simulink model "rate_feedforward_test"  (R2018b)
settings: Solver=FixedStepAuto  StartTime=0.0  StopTime=600  FixedStep=simParams.sample_time_s  RelTol=1e-3
undefined symbols (not defined in the file): simParams
libraries: aerolibutil x2, simulink x1, vrlib x1, clock_lib x1, groundpass_predict_lib x1, sgp4_lib_fsw x1, sunVectorEclipse_lib x1, time_coord_rotations_lib x1, target_gen_lib x1
settings Model: Creator=Taylor  LastModifiedBy=Taylor

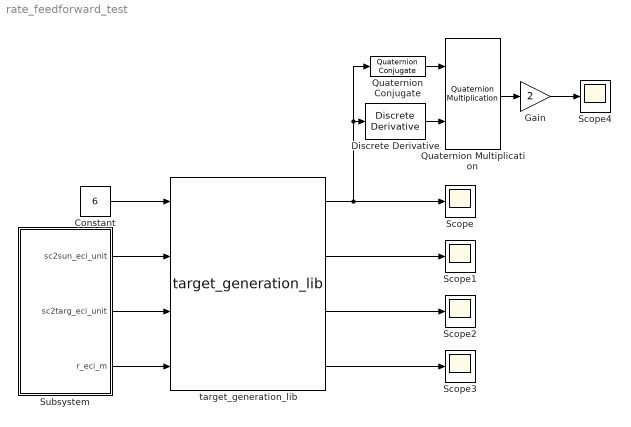
== system rate_feedforward_test ==
  Constant : Constant  Value=6
  Discrete Derivative : simulink/Discrete/Discrete Derivative  gainval=1.0  ICPrevScaledInput=0.0  OutMin=[]  OutMax=[]  OutDataType=fixdt(1, 16)  OutScaling=2^-10  DoSatur=off
  Gain : Gain  Gain=2
  Quaternion Conjugate : aerolibutil/Quaternion Conjugate
      settings: SourceProductName=Aerospace Blockset  SourceProductBaseCode=AE
  Quaternion Multiplication : aerolibutil/Quaternion Multiplication
  Scope{,1..4} (5 alike) : Scope
  Subsystem : Subsystem
  target_generation_lib : target_gen_lib/target_generation_lib  SystemSampleTime=-1
  wires:
  Subsystem/2(sc2targ_eci_unit) -> target_generation_lib/3
  Subsystem/3(r_eci_m) -> target_generation_lib/4
  Subsystem/1(sc2sun_eci_unit) -> target_generation_lib/2
  Constant/1 -> target_generation_lib/1
  target_generation_lib/1 -> Discrete Derivative/1, Quaternion Conjugate/1, Scope/1
  target_generation_lib/2 -> Scope1/1
  target_generation_lib/3 -> Scope2/1
  target_generation_lib/4 -> Scope3/1
  Discrete Derivative/1 -> Quaternion Multiplication/2
  Quaternion Conjugate/1 -> Quaternion Multiplication/1
  Quaternion Multiplication/1 -> Gain/1
  Gain/1 -> Scope4/1

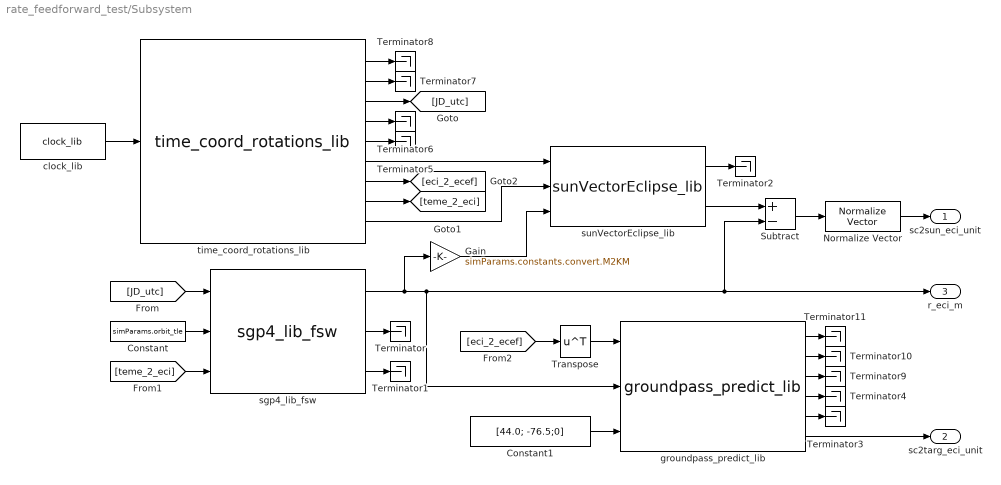
== system rate_feedforward_test/Subsystem ==
  Constant : Constant  Value=simParams.orbit_tle
  Constant1 : Constant  Value=[44.0; -76.5;0]
  Gain : Gain  Gain=simParams.constants.convert.M2KM
  Normalize Vector : vrlib/Utilities/Normalize Vector  maxzero=0
      settings: SourceProductName=Simulink 3D Animation  SourceProductBaseCode=VR
  Subtract : Sum  Inputs=+-
  Terminator{,1..11} (12 alike) : Terminator
  Transpose : Math  Operator=transpose  SaturateOnIntegerOverflow=on
  clock_lib : clock_lib/clock_lib  SystemSampleTime=-1
  groundpass_predict_lib : groundpass_predict_lib/groundpass_predict_lib  SystemSampleTime=-1
  sgp4_lib_fsw : sgp4_lib_fsw/sgp4_lib_fsw  SystemSampleTime=-1
  sunVectorEclipse_lib : sunVectorEclipse_lib/sunVectorEclipse_lib  SystemSampleTime=-1
  "time_coord_rotations_lib " : time_coord_rotations_lib/time_coord_rotations_lib    SystemSampleTime=-1
  sc2sun_eci_unit : Outport
  sc2targ_eci_unit : Outport  Port=2
  r_eci_m : Outport  Port=3
  wires:
  Constant/1 -> sgp4_lib_fsw/2
  clock_lib/1 -> "time_coord_rotations_lib "/1
  [JD_utc] -> sgp4_lib_fsw/1
  [teme_2_eci] -> sgp4_lib_fsw/3
  sgp4_lib_fsw/1 -> Gain/1, groundpass_predict_lib/2, Subtract/2, r_eci_m/1
  sgp4_lib_fsw/2 -> Terminator/1
  sgp4_lib_fsw/3 -> Terminator1/1
  "time_coord_rotations_lib "/3 -> [JD_utc]
  "time_coord_rotations_lib "/9 -> sunVectorEclipse_lib/2
  "time_coord_rotations_lib "/7 -> [eci_2_ecef]
  "time_coord_rotations_lib "/6 -> sunVectorEclipse_lib/1
  "time_coord_rotations_lib "/5 -> Terminator5/1
  "time_coord_rotations_lib "/4 -> Terminator6/1
  "time_coord_rotations_lib "/2 -> Terminator7/1
  "time_coord_rotations_lib "/1 -> Terminator8/1
  "time_coord_rotations_lib "/8 -> [teme_2_eci]
  Gain/1 -> sunVectorEclipse_lib/3
  sunVectorEclipse_lib/2 -> Subtract/1
  Subtract/1 -> Normalize Vector/1
  Normalize Vector/1 -> sc2sun_eci_unit/1
  sunVectorEclipse_lib/1 -> Terminator2/1
  [eci_2_ecef] -> Transpose/1
  Transpose/1 -> groundpass_predict_lib/1
  Constant1/1 -> groundpass_predict_lib/3
  groundpass_predict_lib/6 -> sc2targ_eci_unit/1
  groundpass_predict_lib/5 -> Terminator3/1
  groundpass_predict_lib/4 -> Terminator4/1
  groundpass_predict_lib/3 -> Terminator9/1
  groundpass_predict_lib/2 -> Terminator10/1
  groundpass_predict_lib/1 -> Terminator11/1
